simulink subsystem "earth_horizon_sensor"  (R2023b)
settings: Solver=VariableStepAuto  StartTime=0.0  StopTime=10.0  RelTol=1e-3
undefined symbols (not defined in the file): sensor_data
settings Model: Creator=pierb  LastModifiedBy=Pier Francesco

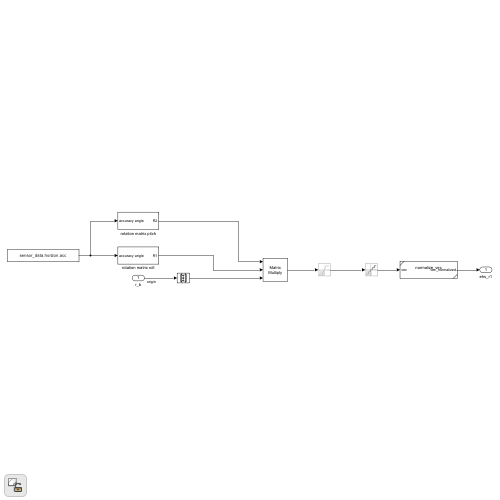
[thumbnail: Simulink's stored preview of the top-level diagram]
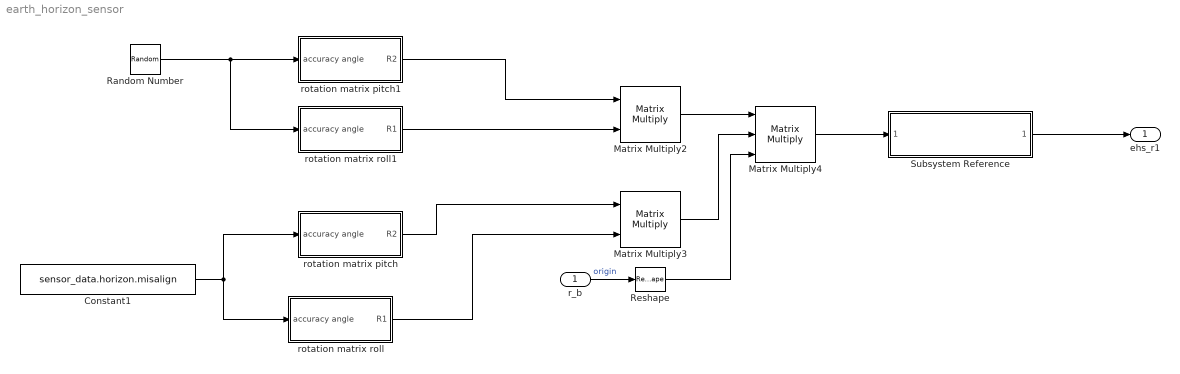
== system earth_horizon_sensor ==
  r_b : Inport
  Constant1 : Constant  Value=sensor_data.horizon.misalign
  Matrix Multiply2 : Product  Multiplication=Matrix(*)
  Matrix Multiply3 : Product  Multiplication=Matrix(*)
  Matrix Multiply4 : Product  Inputs=3  Multiplication=Matrix(*)
  Random Number : RandomNumber  Variance=sensor_data.horizon.acc^2  SampleTime=0.1
  Reshape : Reshape  OutputDimensionality=Column vector (2-D)
  Subsystem Reference : Subsystem  ReferencedSubsystem=normalize_vec
  rotation matrix pitch : Subsystem
  rotation matrix pitch1 : Subsystem
  rotation matrix roll : Subsystem
  rotation matrix roll1 : Subsystem
  ehs_r1 : Outport
  wires:
  Constant1/1 -> rotation matrix pitch/1("accuracy angle "), rotation matrix roll/1("accuracy angle ")
  rotation matrix pitch/1(R2) -> Matrix Multiply3/1
  rotation matrix roll/1(R1) -> Matrix Multiply3/2
  r_b/1 -> Reshape/1  "origin"
  Reshape/1 -> Matrix Multiply4/3
  Subsystem Reference/1 -> ehs_r1/1
  Random Number/1 -> rotation matrix pitch1/1("accuracy angle "), rotation matrix roll1/1("accuracy angle ")
  rotation matrix pitch1/1(R2) -> Matrix Multiply2/1
  rotation matrix roll1/1(R1) -> Matrix Multiply2/2
  Matrix Multiply2/1 -> Matrix Multiply4/1
  Matrix Multiply3/1 -> Matrix Multiply4/2
  Matrix Multiply4/1 -> Subsystem Reference/1

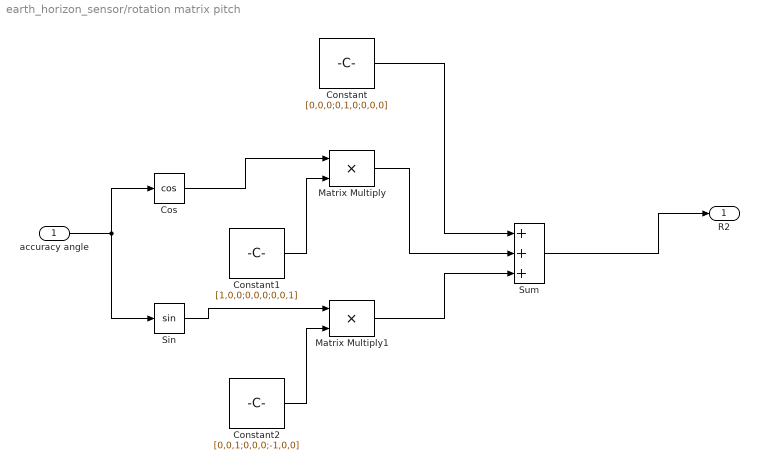
== system earth_horizon_sensor/rotation matrix pitch ==
  "accuracy angle " : Inport
  Constant : Constant  Value=[0,0,0;0,1,0;0,0,0]
  Constant1 : Constant  Value=[1,0,0;0,0,0;0,0,1]
  Constant2 : Constant  Value=[0,0,1;0,0,0;-1,0,0]
  Cos : Trigonometry  Operator=cos
  Matrix Multiply : Product
  Matrix Multiply1 : Product
  Sin : Trigonometry
  Sum : Sum  Inputs=+++
  R2 : Outport
  wires:
  Constant2/1 -> Matrix Multiply1/2
  Sum/1 -> R2/1
  Constant1/1 -> Matrix Multiply/2
  Constant/1 -> Sum/1
  Matrix Multiply1/1 -> Sum/3
  Cos/1 -> Matrix Multiply/1
  Matrix Multiply/1 -> Sum/2
  Sin/1 -> Matrix Multiply1/1
  "accuracy angle "/1 -> Cos/1, Sin/1

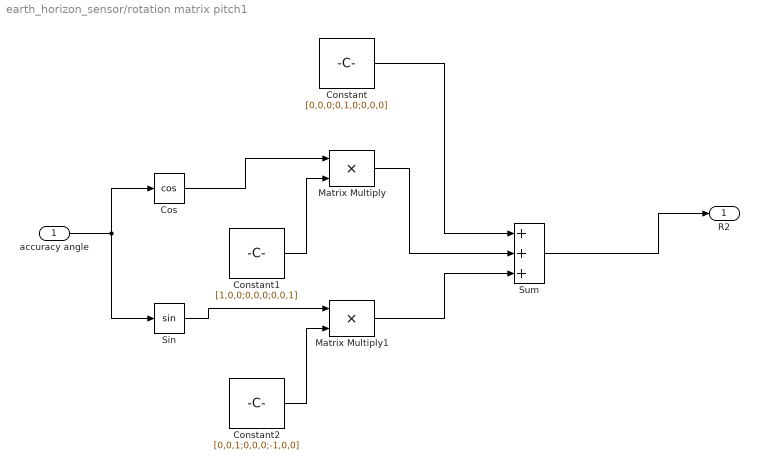
== system earth_horizon_sensor/rotation matrix pitch1 ==
  "accuracy angle " : Inport
  Constant : Constant  Value=[0,0,0;0,1,0;0,0,0]
  Constant1 : Constant  Value=[1,0,0;0,0,0;0,0,1]
  Constant2 : Constant  Value=[0,0,1;0,0,0;-1,0,0]
  Cos : Trigonometry  Operator=cos
  Matrix Multiply : Product
  Matrix Multiply1 : Product
  Sin : Trigonometry
  Sum : Sum  Inputs=+++
  R2 : Outport
  wires:
  "accuracy angle "/1 -> Sin/1, Cos/1
  Sin/1 -> Matrix Multiply1/1
  Matrix Multiply/1 -> Sum/2
  Cos/1 -> Matrix Multiply/1
  Matrix Multiply1/1 -> Sum/3
  Constant/1 -> Sum/1
  Constant1/1 -> Matrix Multiply/2
  Sum/1 -> R2/1
  Constant2/1 -> Matrix Multiply1/2

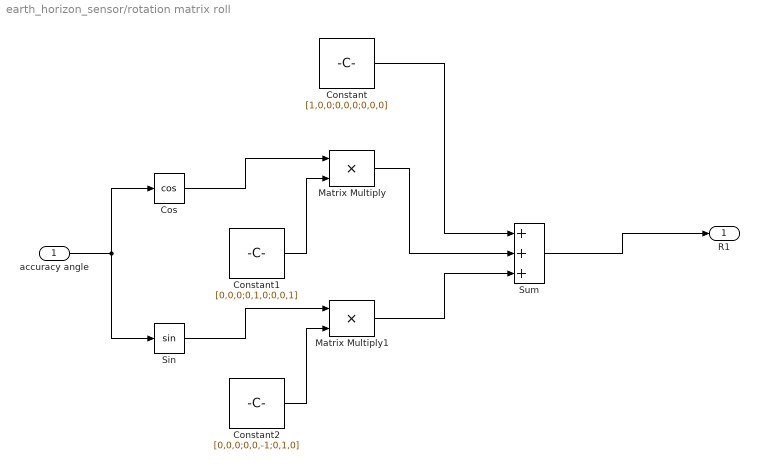
== system earth_horizon_sensor/rotation matrix roll ==
  "accuracy angle " : Inport
  Constant : Constant  Value=[1,0,0;0,0,0;0,0,0]
  Constant1 : Constant  Value=[0,0,0;0,1,0;0,0,1]
  Constant2 : Constant  Value=[0,0,0;0,0,-1;0,1,0]
  Cos : Trigonometry  Operator=cos
  Matrix Multiply : Product
  Matrix Multiply1 : Product
  Sin : Trigonometry
  Sum : Sum  Inputs=+++
  R1 : Outport
  wires:
  Sum/1 -> R1/1
  Matrix Multiply1/1 -> Sum/3
  Matrix Multiply/1 -> Sum/2
  Constant/1 -> Sum/1
  Sin/1 -> Matrix Multiply1/1
  Constant2/1 -> Matrix Multiply1/2
  Cos/1 -> Matrix Multiply/1
  Constant1/1 -> Matrix Multiply/2
  "accuracy angle "/1 -> Cos/1, Sin/1

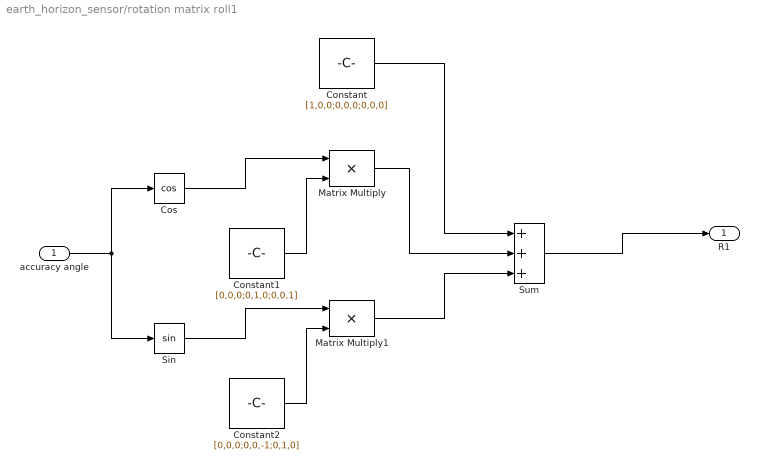
== system earth_horizon_sensor/rotation matrix roll1 ==
  "accuracy angle " : Inport
  Constant : Constant  Value=[1,0,0;0,0,0;0,0,0]
  Constant1 : Constant  Value=[0,0,0;0,1,0;0,0,1]
  Constant2 : Constant  Value=[0,0,0;0,0,-1;0,1,0]
  Cos : Trigonometry  Operator=cos
  Matrix Multiply : Product
  Matrix Multiply1 : Product
  Sin : Trigonometry
  Sum : Sum  Inputs=+++
  R1 : Outport
  wires:
  "accuracy angle "/1 -> Sin/1, Cos/1
  Constant1/1 -> Matrix Multiply/2
  Cos/1 -> Matrix Multiply/1
  Constant2/1 -> Matrix Multiply1/2
  Sin/1 -> Matrix Multiply1/1
  Constant/1 -> Sum/1
  Matrix Multiply/1 -> Sum/2
  Matrix Multiply1/1 -> Sum/3
  Sum/1 -> R1/1
